simulink model "basic_template_project"  (R2015b)
settings: Solver=VariableStepAuto  StartTime=0.0  StopTime=10.0  RelTol=1e-3
settings Model: Creator=GusBus  LastModifiedBy=GusBus

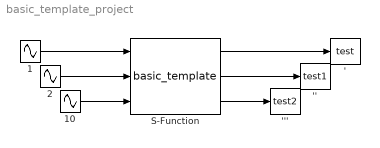
== system basic_template_project ==
  ' : ToWorkspace  VariableName=test  SaveFormat=Timeseries  SampleTime=-1
  '' : ToWorkspace  VariableName=test1  SaveFormat=Timeseries  SampleTime=-1
  ''' : ToWorkspace  VariableName=test2  SaveFormat=Timeseries  SampleTime=-1
  1 : Sin  SampleTime=0
  10 : Sin  Amplitude=10  SampleTime=0
  2 : Sin  Amplitude=2  SampleTime=0
  S-Function : S-Function  FunctionName=basic_template  SFunctionDeploymentMode=off  EnableBusSupport=off
  wires:
  1/1 -> S-Function/1
  2/1 -> S-Function/2
  10/1 -> S-Function/3
  S-Function/1 -> '/1
  S-Function/3 -> '''/1
  S-Function/2 -> ''/1
